simulink model "quadplane_control_conf"  (R2023a)
settings: Solver=FixedStepAuto  StartTime=0.0  StopTime=10.0  FixedStep=0.001  RelTol=1e-3
undefined symbols (not defined in the file or in its folder): Aircraft, DiscIntNeverNeededParam, framePeriod_s, frameRate_hz
libraries: simulink x14, fuzblock x1
(part 1 of 2)
settings Model: Creator=lagerprocessor  LastModifiedBy=abhandari1
settings DebuggingCC: ParameterPrecisionLossMsg=none

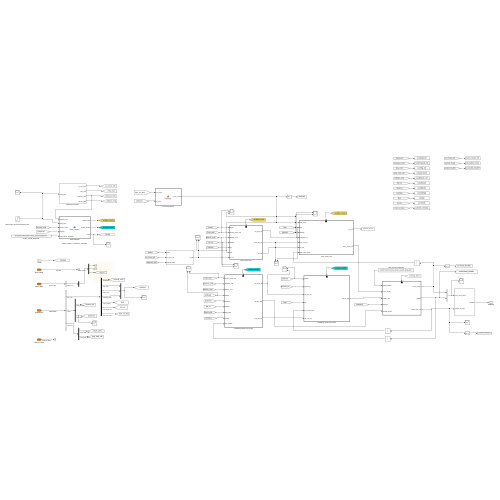
[thumbnail: Simulink's stored preview of the top-level diagram]
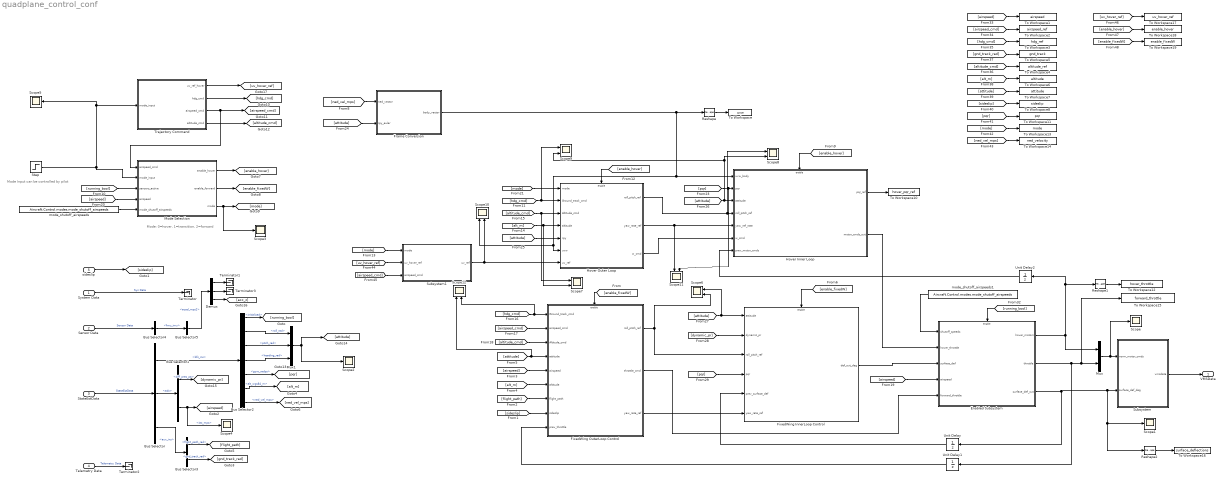
== system quadplane_control_conf ==
  note: Mode Input can be controlled by pilot
  note: Mode: 0=hover, 1=transition, 2=forward
  System Data : Inport  OutDataTypeStr=Bus: SysData  SampleTime=framePeriod_s  BusOutputAsStruct=on
  Sensor Data : Inport  Port=2  OutDataTypeStr=Bus: SensorData  SampleTime=framePeriod_s  BusOutputAsStruct=on
  StateEstData : Inport  Port=3  OutDataTypeStr=Bus: StateEstData  BusOutputAsStruct=on
  Telemetry Data : Inport  Port=4  OutDataTypeStr=Bus: TelemData  SampleTime=framePeriod_s  BusOutputAsStruct=on
  sideslip : Inport  Port=5  OutDataTypeStr=single
  Bus Selector : BusSelector  OutputSignals=bfs_ins,adc,aux_ins
  Bus Selector1 : BusSelector  OutputSignals=diff_pres_pa,ias_mps
  Bus Selector2 : BusSelector  OutputSignals=initialized,roll_rad,pitch_rad,heading_rad,gyro_radps,alt_wgs84_m,ned_vel_mps
  Bus Selector3 : BusSelector  OutputSignals=flight_path_rad,gnd_track_rad
  Bus Selector4 : BusSelector  OutputSignals=fmu_imu
  Bus Selector5 : BusSelector  OutputSignals=accel_mps2
  Demux : Demux  Outputs=3
  Enabled Subsystem : Subsystem  TreatAsAtomicUnit=on
  FixedWing InnerLoop Control : Subsystem  TreatAsAtomicUnit=on
  FixedWing OuterLoop Control : Subsystem  TreatAsAtomicUnit=on
  Frame Conversion : MATLAB Function  TreatAsAtomicUnit=on
  Hover Inner Loop : Subsystem  TreatAsAtomicUnit=on
  Hover Outer Loop : Subsystem  TreatAsAtomicUnit=on
  Mode Selection : MATLAB Function  TreatAsAtomicUnit=on
  Mux : Mux  Inputs=2
  Mux1 : Mux  Inputs=3
  Reshape : Reshape
  Reshape1 : Reshape
  Reshape2 : Reshape
  Scope{,1..5} (6 alike) : Scope
  Scope{6..12} (7 alike) : Scope  NumInputPorts=2
  Step : Step  Time=7  OutDataTypeStr=single  SampleTime=0
  Subsystem : Subsystem
  Subsystem1 : Subsystem
  Terminator{,1..3} (4 alike) : Terminator
  To Workspace : ToWorkspace  VariableName=uvw  SampleTime=-1
      settings: Save2DSignal=2-D array (concatenate along first dimension)
  To Workspace1 : ToWorkspace  VariableName=airspeed  SaveFormat=Timeseries  SampleTime=-1
  To Workspace10 : ToWorkspace  VariableName=hover_pqr_ref  SaveFormat=Timeseries  SampleTime=-1
  To Workspace11 : ToWorkspace  VariableName=pqr  SaveFormat=Timeseries  SampleTime=-1
  To Workspace12 : ToWorkspace  VariableName=hover_throttle  SampleTime=-1
      settings: Save2DSignal=2-D array (concatenate along first dimension)
  To Workspace13 : ToWorkspace  VariableName=mode  SaveFormat=Timeseries  SampleTime=-1
  To Workspace14 : ToWorkspace  VariableName=ned_velocity  SaveFormat=Timeseries  SampleTime=-1
  To Workspace15 : ToWorkspace  VariableName=forward_throttle  SaveFormat=Timeseries  SampleTime=-1
  To Workspace16 : ToWorkspace  VariableName=surface_deflections  SampleTime=-1
      settings: Save2DSignal=2-D array (concatenate along first dimension)
  To Workspace17 : ToWorkspace  VariableName=uv_hover_ref  SaveFormat=Timeseries  SampleTime=-1
  To Workspace18 : ToWorkspace  VariableName=enable_hover  SaveFormat=Timeseries  SampleTime=-1
  To Workspace19 : ToWorkspace  VariableName=enable_fixedW  SaveFormat=Timeseries  SampleTime=-1
  To Workspace2 : ToWorkspace  VariableName=airspeed_ref  SaveFormat=Timeseries  SampleTime=-1
  To Workspace3 : ToWorkspace  VariableName=hdg_ref  SaveFormat=Timeseries  SampleTime=-1
  To Workspace4 : ToWorkspace  VariableName=altitude_ref  SaveFormat=Timeseries  SampleTime=-1
  To Workspace5 : ToWorkspace  VariableName=gnd_track  SaveFormat=Timeseries  SampleTime=-1
  To Workspace6 : ToWorkspace  VariableName=altitude  SaveFormat=Timeseries  SampleTime=-1
  To Workspace7 : ToWorkspace  VariableName=attitude  SaveFormat=Timeseries  SampleTime=-1
  To Workspace8 : ToWorkspace  VariableName=sideslip  SaveFormat=Timeseries  SampleTime=-1
  Trajectory Command : Subsystem
  Unit Delay : UnitDelay  SampleTime=-1  HasFrameUpgradeWarning=on
  Unit Delay1 : UnitDelay  SampleTime=-1  HasFrameUpgradeWarning=on
  Unit Delay2 : UnitDelay  SampleTime=-1  HasFrameUpgradeWarning=on
  mode_shutoff_airspeeds : Constant  Value=Aircraft.Control.modes.mode_shutoff_airspeeds  OutDataTypeStr=single
  mode_shutoff_airspeeds1 : Constant  Value=Aircraft.Control.modes.mode_shutoff_airspeeds  OutDataTypeStr=single
  VMSData : Outport  OutDataTypeStr=Bus: VmsData
  wires:
  Telemetry Data/1 -> Terminator2/1  "Telemetry Data"
  StateEstData/1 -> Bus Selector/1  "StateEstData"
  Sensor Data/1 -> Bus Selector4/1  "Sensor Data"
  System Data/1 -> Terminator/1  "Sys Data"
  Subsystem/1(vmsdata) -> VMSData/1
  Bus Selector/2 -> Bus Selector1/1  "<adc>"
  Bus Selector/1 -> Bus Selector2/1  "<bfs_ins>"
  [enable_fixedW] -> FixedWing InnerLoop Control/Enable
  Bus Selector2/3 -> Mux1/2  "<pitch_rad>"
  Bus Selector2/4 -> Mux1/3  "<heading_rad>"
  Bus Selector/3 -> Bus Selector3/1  "<aux_ins>"
  Bus Selector4/1 -> Bus Selector5/1  "<fmu_imu>"
  Bus Selector5/1 -> Demux/1  "<accel_mps2>"
  Demux/1 -> Terminator1/1
  Demux/2 -> Terminator3/1
  sideslip/1 -> [sideslip]
  [sideslip] -> FixedWing OuterLoop Control/8(sideslip)
  Bus Selector2/1 -> [running_bool]  "<initialized>"
  Bus Selector2/2 -> Mux1/1  "<roll_rad>"
  [hdg_cmd] -> Scope12/2, FixedWing OuterLoop Control/1(Ground_track_cmd)
  Bus Selector3/2 -> [gnd_track_rad]  "<gnd_track_rad>"
  Bus Selector2/6 -> [alt_m]  "<alt_wgs84_m>"
  FixedWing OuterLoop Control/1(roll_pitch_ref) -> FixedWing InnerLoop Control/3(roll_pitch_ref), Scope6/2
  [airspeed_cmd] -> FixedWing OuterLoop Control/2(airspeed_cmd)
  [altitude_cmd] -> FixedWing OuterLoop Control/3(Altitude_cmd)
  [flight_path] -> FixedWing OuterLoop Control/7(flight_path)
  [airspeed] -> FixedWing OuterLoop Control/5(airspeed)
  [alt_m] -> FixedWing OuterLoop Control/6(altitude)
  [attitude] -> Scope12/1, FixedWing OuterLoop Control/4(attitude)
  [enable_fixedW] -> FixedWing OuterLoop Control/Enable
  Bus Selector2/7 -> [ned_vel_mps]  "<ned_vel_mps>"
  [ned_vel_mps] -> Frame Conversion/1(ned_vector)
  FixedWing OuterLoop Control/2(throttle_cmd) -> Enabled Subsystem/5(forward_throttle)
  FixedWing InnerLoop Control/1(def_out_deg) -> Enabled Subsystem/3(surface_def)
  [enable_hover] -> Hover Inner Loop/Enable
  Hover Inner Loop/2(motor_cmds_out) -> Enabled Subsystem/2(hover_throttle)
  Hover Outer Loop/1(roll_pitch_ref) -> Scope8/1, Hover Inner Loop/4(roll_pitch_ref)
  Hover Outer Loop/2(yaw_rate_ref) -> Hover Inner Loop/5(yaw_ref_rate), Scope11/1
  [enable_hover] -> Hover Outer Loop/Enable
  Hover Outer Loop/3(w_cmd) -> Hover Inner Loop/6(w_cmd)
  [hdg_cmd] -> Scope9/1, Hover Outer Loop/2(Ground_track_cmd)
  [altitude_cmd] -> Scope7/1, Hover Outer Loop/3(Altitude_cmd)
  [alt_m] -> Hover Outer Loop/4(altitude), Scope7/2
  Step/1 -> Mode Selection/2(mode_input), Scope5/1, Trajectory Command/1(mode_input)
  Mode Selection/1(enable_hover) -> [enable_hover]
  Mode Selection/2(enable_forward) -> [enable_fixedW]
  [running_bool] -> Mode Selection/3(sensors_active)
  Trajectory Command/2(hdg_cmd) -> [hdg_cmd]
  Trajectory Command/4(altitude_cmd) -> [altitude_cmd]
  Trajectory Command/3(airspeed_cmd) -> [airspeed_cmd], Mode Selection/1(airspeed_cmd)
  [airspeed] -> Enabled Subsystem/4(airspeed)
  Mux/1 -> Scope/1, Subsystem/1(norm_motor_cmds)
  Enabled Subsystem/2(throttle) -> Unit Delay1/1, To Workspace15/1, Mux/2
  Unit Delay/1 -> FixedWing InnerLoop Control/5(prev_surface_def)
  Unit Delay1/1 -> FixedWing OuterLoop Control/9(prev_throttle)
  Unit Delay2/1 -> Hover Inner Loop/7(prev_motor_cmds)
  [airspeed] -> Mode Selection/4(airspeed)
  mode_shutoff_airspeeds/1 -> Mode Selection/5(mode_shutoff_airspeeds)
  [mode] -> Hover Outer Loop/1(mode)
  Mode Selection/3(mode) -> Scope3/1, [mode]
  Bus Selector2/5 -> [pqr]  "<gyro_radps>"
  Mux1/1 -> Scope2/1, [attitude]
  Bus Selector1/1 -> [dynamic_pr]  "<diff_pres_pa>"
  Bus Selector3/1 -> [flight_path]  "<flight_path_rad>"
  Demux/3 -> [acc_z]
  [attitude] -> Frame Conversion/2(rpy_euler)
  [attitude] -> Hover Outer Loop/5(rpy)
  [pqr] -> Scope11/2, Hover Inner Loop/2(pqr)
  [attitude] -> Scope8/2, Scope9/2, Hover Inner Loop/3(attitude)
  [attitude] -> Scope6/1, FixedWing InnerLoop Control/1(attitude)
  [dynamic_pr] -> FixedWing InnerLoop Control/2(dynamic_pr)
  [pqr] -> FixedWing InnerLoop Control/4(pqr)
  mode_shutoff_airspeeds1/1 -> Enabled Subsystem/1(shutoff_speeds)
  Bus Selector1/2 -> Scope4/1, [airspeed]  "<ias_mps>"
  [running_bool] -> Enabled Subsystem/Enable
  Frame Conversion/1(body_vector) -> Reshape/1, Scope10/1, Hover Outer Loop/6(uvw), Hover Inner Loop/1(uvw_body)
  [airspeed] -> To Workspace1/1
  [airspeed_cmd] -> To Workspace2/1
  [hdg_cmd] -> To Workspace3/1
  [altitude_cmd] -> To Workspace4/1
  [gnd_track_rad] -> To Workspace5/1
  [alt_m] -> To Workspace6/1
  [attitude] -> To Workspace7/1
  [sideslip] -> To Workspace8/1
  Hover Inner Loop/1(pqr_ref) -> To Workspace10/1
  [pqr] -> To Workspace11/1
  [mode] -> To Workspace13/1
  [ned_vel_mps] -> To Workspace14/1
  Trajectory Command/1(uv_ref_hover) -> [uv_hover_ref]
  Reshape/1 -> To Workspace/1
  Enabled Subsystem/1(hover_motors) -> Mux/1, Reshape1/1, Unit Delay2/1
  Reshape1/1 -> To Workspace12/1
  Enabled Subsystem/3(surface_def_out) -> Scope1/1, Reshape2/1, Subsystem/2(surface_def_deg), Unit Delay/1
  Reshape2/1 -> To Workspace16/1
  Subsystem1/1(uv_ref) -> Scope10/2, Hover Outer Loop/7(uv_ref)
  [mode] -> Subsystem1/1(mode)
  [airspeed_cmd] -> Subsystem1/3(airspeed_cmd)
  [uv_hover_ref] -> Subsystem1/2(uv_hover_ref)
  [enable_hover] -> To Workspace18/1
  [enable_fixedW] -> To Workspace19/1
  [uv_hover_ref] -> To Workspace17/1
  FixedWing OuterLoop Control/3(yaw_rate_ref) -> FixedWing InnerLoop Control/6(yaw_rate_ref)

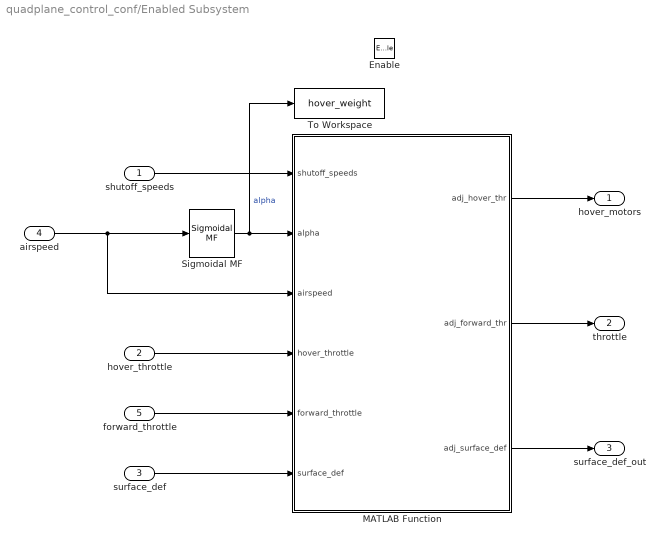
== system quadplane_control_conf/Enabled Subsystem ==
  shutoff_speeds : Inport
  hover_throttle : Inport  Port=2
  surface_def : Inport  Port=3
  airspeed : Inport  Port=4
  forward_throttle : Inport  Port=5
  Enable : EnablePort
  MATLAB Function : MATLAB Function  TreatAsAtomicUnit=on
  Sigmoidal MF : fuzblock/Membership  Functions/Sigmoidal MF  a=Aircraft.Control.modes.transition_sigmoidal_a  c=Aircraft.Control.modes.transition_sigmoidal_c
  To Workspace : ToWorkspace  VariableName=hover_weight  SaveFormat=Timeseries  SampleTime=-1
  hover_motors : Outport
  throttle : Outport  Port=2
  surface_def_out : Outport  Port=3
  wires:
  MATLAB Function/3(adj_surface_def) -> surface_def_out/1
  shutoff_speeds/1 -> MATLAB Function/1(shutoff_speeds)
  MATLAB Function/2(adj_forward_thr) -> throttle/1
  airspeed/1 -> MATLAB Function/3(airspeed), Sigmoidal MF/1
  forward_throttle/1 -> MATLAB Function/5(forward_throttle)
  surface_def/1 -> MATLAB Function/6(surface_def)
  Sigmoidal MF/1 -> To Workspace/1, MATLAB Function/2(alpha)  "alpha"
  MATLAB Function/1(adj_hover_thr) -> hover_motors/1
  hover_throttle/1 -> MATLAB Function/4(hover_throttle)

== system quadplane_control_conf/FixedWing InnerLoop Control ==
  attitude : Inport
  dynamic_pr : Inport  Port=2
  roll_pitch_ref : Inport  Port=3
  pqr : Inport  Port=4
  prev_surface_def : Inport  Port=5
  yaw_rate_ref : Inport  Port=6
  Enable : EnablePort
  INDI Based Angular Rate Controller : Subsystem
  NDI based Attitude Controller : Subsystem
  def_out_deg : Outport
  wires:
  dynamic_pr/1 -> INDI Based Angular Rate Controller/1(dynamic_pr)
  pqr/1 -> INDI Based Angular Rate Controller/3(pqr)
  attitude/1 -> NDI based Attitude Controller/1(attitude)
  NDI based Attitude Controller/1(pqr_ref) -> INDI Based Angular Rate Controller/2(pqr_ref)
  roll_pitch_ref/1 -> NDI based Attitude Controller/2(roll_pitch_ref)
  prev_surface_def/1 -> INDI Based Angular Rate Controller/4(prev_surface_def)
  INDI Based Angular Rate Controller/1(def_out_deg) -> def_out_deg/1
  yaw_rate_ref/1 -> NDI based Attitude Controller/3(yaw_rate_ref)

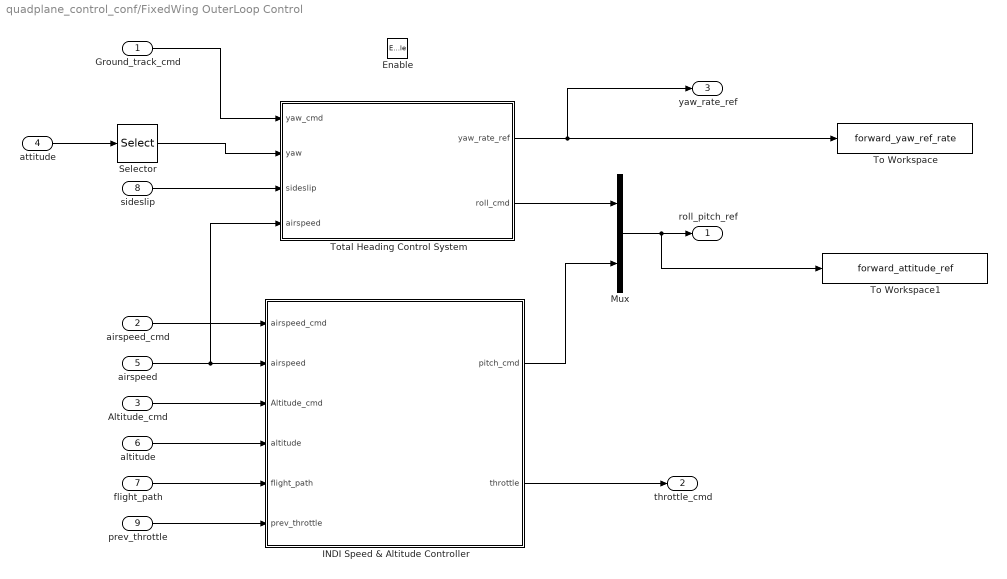
== system quadplane_control_conf/FixedWing OuterLoop Control ==
  Ground_track_cmd : Inport
  airspeed_cmd : Inport  Port=2
  Altitude_cmd : Inport  Port=3
  attitude : Inport  Port=4
  airspeed : Inport  Port=5
  altitude : Inport  Port=6
  flight_path : Inport  Port=7
  sideslip : Inport  Port=8
  prev_throttle : Inport  Port=9
  Enable : EnablePort
  INDI Speed & Altitude Controller : Subsystem
  Mux : Mux  Inputs=2
  Selector : Selector  InputPortWidth=3  IndexOptions=Index vector (dialog)  Indices=3  OutputSizes=1
  To Workspace : ToWorkspace  VariableName=forward_yaw_ref_rate  SaveFormat=Timeseries  SampleTime=-1
  To Workspace1 : ToWorkspace  VariableName=forward_attitude_ref  SaveFormat=Timeseries  SampleTime=-1
  Total Heading Control System : Subsystem
  roll_pitch_ref : Outport
  throttle_cmd : Outport  Port=2
  yaw_rate_ref : Outport  Port=3
  wires:
  Ground_track_cmd/1 -> Total Heading Control System/1(yaw_cmd)
  Altitude_cmd/1 -> INDI Speed & Altitude Controller/3(Altitude_cmd)
  INDI Speed & Altitude Controller/2(throttle) -> throttle_cmd/1
  altitude/1 -> INDI Speed & Altitude Controller/4(altitude)
  flight_path/1 -> INDI Speed & Altitude Controller/5(flight_path)
  INDI Speed & Altitude Controller/1(pitch_cmd) -> Mux/2
  airspeed_cmd/1 -> INDI Speed & Altitude Controller/1(airspeed_cmd)
  Total Heading Control System/2(roll_cmd) -> Mux/1
  airspeed/1 -> Total Heading Control System/4(airspeed), INDI Speed & Altitude Controller/2(airspeed)
  Selector/1 -> Total Heading Control System/2(yaw)
  prev_throttle/1 -> INDI Speed & Altitude Controller/6(prev_throttle)
  Mux/1 -> To Workspace1/1, roll_pitch_ref/1
  attitude/1 -> Selector/1
  sideslip/1 -> Total Heading Control System/3(sideslip)
  Total Heading Control System/1(yaw_rate_ref) -> yaw_rate_ref/1, To Workspace/1

== system quadplane_control_conf/Hover Inner Loop ==
  uvw_body : Inport
  pqr : Inport  Port=2
  attitude : Inport  Port=3
  roll_pitch_ref : Inport  Port=4
  yaw_ref_rate : Inport  Port=5
  w_cmd : Inport  Port=6
  prev_motor_cmds : Inport  Port=7
  Enable : EnablePort
  Attitude Control : Subsystem
  INDI inner loop : Subsystem
  pqr_ref : Outport
  motor_cmds_out : Outport  Port=2
  wires:
  Attitude Control/1(pqr_ref1) -> pqr_ref/1, INDI inner loop/1(pqr_ref)
  uvw_body/1 -> INDI inner loop/2(uvw_body)
  pqr/1 -> INDI inner loop/4(pqr)
  INDI inner loop/1(motor_cmds_out) -> motor_cmds_out/1
  attitude/1 -> Attitude Control/3(roll_pitch_yaw)
  yaw_ref_rate/1 -> Attitude Control/1(yaw_rate_ref)
  roll_pitch_ref/1 -> Attitude Control/2(roll_pitch_ref)
  w_cmd/1 -> INDI inner loop/3(w_ref)
  prev_motor_cmds/1 -> INDI inner loop/5(prev_motor_cmds)

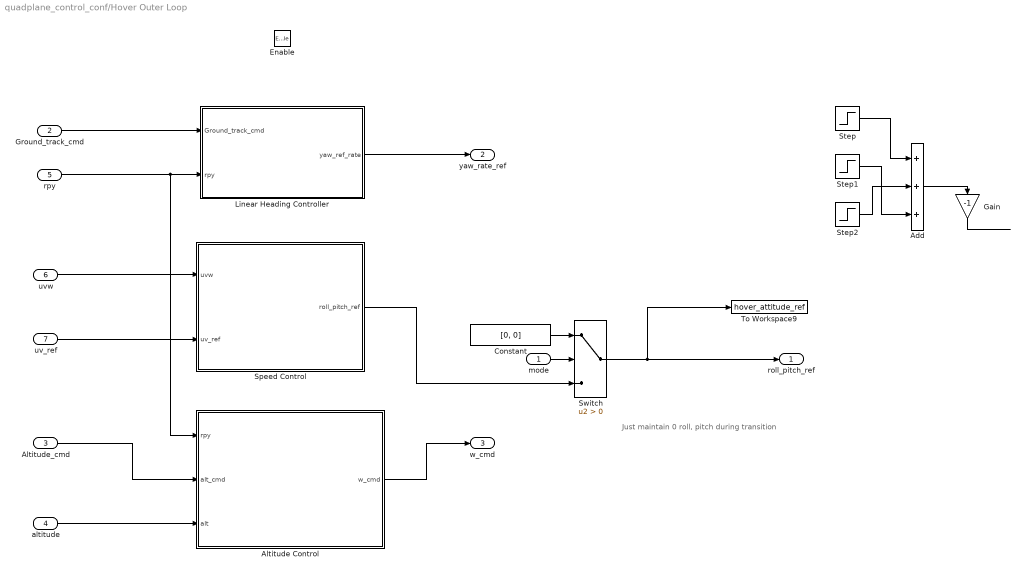
== system quadplane_control_conf/Hover Outer Loop ==
  note: Just maintain 0 roll, pitch during transition
  mode : Inport
  Ground_track_cmd : Inport  Port=2
  Altitude_cmd : Inport  Port=3
  altitude : Inport  Port=4
  rpy : Inport  Port=5
  uvw : Inport  Port=6
  uv_ref : Inport  Port=7
  Enable : EnablePort
  Add : Sum  Inputs=+++
  Altitude Control : Subsystem
  Constant : Constant  Value=[0, 0]  OutDataTypeStr=single
  Gain : Gain  Gain=-1
  Linear Heading Controller : Subsystem
  Speed Control : Subsystem
  Step : Step  Time=2  After=0.5  OutDataTypeStr=single  SampleTime=0
  Step1 : Step  Time=4  Before=0.5  After=-0.5  OutDataTypeStr=single  SampleTime=0
  Step2 : Step  Time=7  Before=-0.5  After=0  OutDataTypeStr=single  SampleTime=0
  Switch : Switch  Criteria=u2 > Threshold  SaturateOnIntegerOverflow=off  InputSameDT=off
  To Workspace9 : ToWorkspace  VariableName=hover_attitude_ref  SaveFormat=Timeseries  SampleTime=-1
  roll_pitch_ref : Outport
  yaw_rate_ref : Outport  Port=2
  w_cmd : Outport  Port=3
  wires:
  Ground_track_cmd/1 -> Linear Heading Controller/1(Ground_track_cmd)
  Altitude_cmd/1 -> Altitude Control/2(alt_cmd)
  altitude/1 -> Altitude Control/3(alt)
  rpy/1 -> Altitude Control/1(rpy), Linear Heading Controller/2(rpy)
  uvw/1 -> Speed Control/1(uvw)
  Speed Control/1(roll_pitch_ref) -> Switch/3
  Altitude Control/1(w_cmd) -> w_cmd/1
  Switch/1 -> To Workspace9/1, roll_pitch_ref/1
  mode/1 -> Switch/2
  Constant/1 -> Switch/1
  uv_ref/1 -> Speed Control/2(uv_ref)
  Step/1 -> Add/1
  Step1/1 -> Add/3
  Step2/1 -> Add/2
  Add/1 -> Gain/1
  Gain/1 -> ?
  Linear Heading Controller/1(yaw_ref_rate) -> yaw_rate_ref/1

== system quadplane_control_conf/Subsystem ==
  note: norm_motor_cmds = [0,1]
  note: surface_def = [-30, 30]
  norm_motor_cmds : Inport
  surface_def_deg : Inport  Port=2
  Subsystem1 : Subsystem
  deflections_PWM_denormalize : Subsystem
  motor_PWM_denormalize : Subsystem
  vmsdata : Outport
  wires:
  motor_PWM_denormalize/1(raw_output) -> Subsystem1/1(Motor_Cmds)
  deflections_PWM_denormalize/1(raw_output) -> Subsystem1/2(Surface_def)
  Subsystem1/1(vmsdata) -> vmsdata/1
  norm_motor_cmds/1 -> motor_PWM_denormalize/1(normalized_input)
  surface_def_deg/1 -> deflections_PWM_denormalize/1(normalized_input)

== system quadplane_control_conf/Subsystem1 ==
  mode : Inport
  uv_hover_ref : Inport  Port=2
  airspeed_cmd : Inport  Port=3
  Constant : Constant  Value=0  OutDataTypeStr=single
  Mux : Mux  Inputs=2
  Switch : Switch  Criteria=u2 > Threshold  SaturateOnIntegerOverflow=off  InputSameDT=off
  uv_ref : Outport
  wires:
  Switch/1 -> uv_ref/1
  mode/1 -> Switch/2
  airspeed_cmd/1 -> Mux/1
  Constant/1 -> Mux/2
  Mux/1 -> Switch/1
  uv_hover_ref/1 -> Switch/3

== system quadplane_control_conf/Trajectory Command ==
  mode_input : Inport
  Subsystem : Subsystem
  Subsystem1 : Subsystem
  Subsystem2 : Subsystem
  Subsystem3 : Subsystem
  uv_ref_hover : Outport
  hdg_cmd : Outport  Port=2
  airspeed_cmd : Outport  Port=3
  altitude_cmd : Outport  Port=4
  wires:
  Subsystem/1(uv_ref_hover) -> uv_ref_hover/1
  Subsystem1/1(hdg_cmd) -> hdg_cmd/1
  Subsystem2/1(airspeed_cmd) -> airspeed_cmd/1
  Subsystem3/1(altitude_cmd) -> altitude_cmd/1
  mode_input/1 -> Subsystem2/1(mode_input)

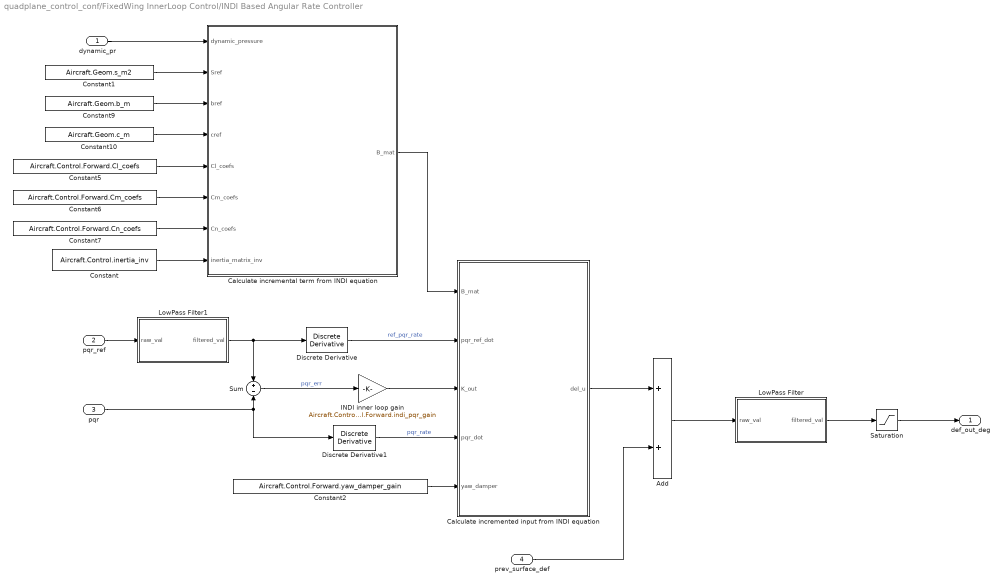
== system quadplane_control_conf/FixedWing InnerLoop Control/INDI Based Angular Rate Controller ==
  dynamic_pr : Inport
  pqr_ref : Inport  Port=2
  pqr : Inport  Port=3
  prev_surface_def : Inport  Port=4
  Add : Sum  OutDataTypeStr=single
  Calculate incremental term from INDI equation : MATLAB Function  TreatAsAtomicUnit=on
  Calculate incremented input from INDI equation : MATLAB Function  TreatAsAtomicUnit=on
  Constant : Constant  Value=Aircraft.Control.inertia_inv  OutDataTypeStr=single
  Constant1 : Constant  Value=Aircraft.Geom.s_m2  OutDataTypeStr=single
  Constant10 : Constant  Value=Aircraft.Geom.c_m  OutDataTypeStr=single
  Constant2 : Constant  Value=Aircraft.Control.Forward.yaw_damper_gain  OutDataTypeStr=single
  Constant5 : Constant  Value=Aircraft.Control.Forward.Cl_coefs  OutDataTypeStr=single
  Constant6 : Constant  Value=Aircraft.Control.Forward.Cm_coefs  OutDataTypeStr=single
  Constant7 : Constant  Value=Aircraft.Control.Forward.Cn_coefs  OutDataTypeStr=single
  Constant9 : Constant  Value=Aircraft.Geom.b_m  OutDataTypeStr=single
  Discrete Derivative : simulink/Discrete/Discrete Derivative  gainval=1.0  ICPrevScaledInput=0.0  OutMin=[]  OutMax=[]  OutDataTypeStr=single  OutputDataTypeScalingMode=single  OutDataType=fixdt(1, 16)  OutScaling=2^-10  DoSatur=off
  Discrete Derivative1 : simulink/Discrete/Discrete Derivative  gainval=1.0  ICPrevScaledInput=0.0  OutMin=[]  OutMax=[]  OutDataType=fixdt(1, 16)  OutScaling=2^-10  DoSatur=off
  INDI inner loop gain : Gain  Gain=Aircraft.Control.Forward.indi_pqr_gain  OutDataTypeStr=single
  LowPass Filter : Subsystem
      settings: PortSchema="{\"entries\":[{\"content\":{\"sides\":[{\"content\":{\"connectorIds\":[\"Out1\"]},\"type\":\"ConnectorPlacement.EquallySpacedRectSide\",\"uuid\":\"91cc3e13-2b14-472d-8884-d1975898cd34\"},{\"content\":{\"connectorIds\":[\"In1\"],\"side\":\"RIGHT\"},\"type\":\"ConnectorPlacement.EquallySpacedRectSide\",\"uuid\":\"ce6b3021-6e32-4737-8c8e-25014706d3dd\"},{\"content\":{\"side\":\"TOP\"},\"type\":\"ConnectorPlacement.EquallySpacedRectSide\",\"uuid\":\"ad734f0b-b067-43e6-a641-0e0955250a7f\"},{\"content\":{\"side\":\"BOTTOM\"},\"type\":\"ConnectorPlacement.EquallySpacedRectSide\",\"uuid\":\"618c62c8-d4e2-4678-9fe1-905e2f147d5d\"}]},\"type\":\"ConnectorPlacement.EquallySpacedConnector\",\"uuid\":\"c0097053-d36a-473a-84fb-0616f69f4bc5\"}],\"packageUris\":[\"http://schema.mathworks.com/mf0/Connector/R2020b\"],\"version\":\"1.0\"}"
  LowPass Filter1 : Subsystem
      settings: PortSchema="{\"entries\":[{\"content\":{\"sides\":[{\"content\":{\"connectorIds\":[\"Out1\"]},\"type\":\"ConnectorPlacement.EquallySpacedRectSide\",\"uuid\":\"91cc3e13-2b14-472d-8884-d1975898cd34\"},{\"content\":{\"connectorIds\":[\"In1\"],\"side\":\"RIGHT\"},\"type\":\"ConnectorPlacement.EquallySpacedRectSide\",\"uuid\":\"ce6b3021-6e32-4737-8c8e-25014706d3dd\"},{\"content\":{\"side\":\"TOP\"},\"type\":\"ConnectorPlacement.EquallySpacedRectSide\",\"uuid\":\"ad734f0b-b067-43e6-a641-0e0955250a7f\"},{\"content\":{\"side\":\"BOTTOM\"},\"type\":\"ConnectorPlacement.EquallySpacedRectSide\",\"uuid\":\"618c62c8-d4e2-4678-9fe1-905e2f147d5d\"}]},\"type\":\"ConnectorPlacement.EquallySpacedConnector\",\"uuid\":\"c0097053-d36a-473a-84fb-0616f69f4bc5\"}],\"packageUris\":[\"http://schema.mathworks.com/mf0/Connector/R2020b\"],\"version\":\"1.0\"}"
  Saturation : Saturate  UpperLimit=Aircraft.Surf.Limit.pos_deg  LowerLimit=Aircraft.Surf.Limit.neg_deg  OutDataTypeStr=single
  Sum : Sum  Inputs=+-
  def_out_deg : Outport
  wires:
  Discrete Derivative1/1 -> Calculate incremented input from INDI equation/4(pqr_dot)  "pqr_rate"
  Constant2/1 -> Calculate incremented input from INDI equation/5(yaw_damper)
  Constant7/1 -> Calculate incremental term from INDI equation/7(Cn_coefs)
  Discrete Derivative/1 -> Calculate incremented input from INDI equation/2(pqr_ref_dot)  "ref_pqr_rate"
  Saturation/1 -> def_out_deg/1
  dynamic_pr/1 -> Calculate incremental term from INDI equation/1(dynamic_pressure)
  Constant1/1 -> Calculate incremental term from INDI equation/2(Sref)
  Constant10/1 -> Calculate incremental term from INDI equation/4(cref)
  Calculate incremented input from INDI equation/1(del_u) -> Add/1
  Constant6/1 -> Calculate incremental term from INDI equation/6(Cm_coefs)
  Sum/1 -> INDI inner loop gain/1  "pqr_err"
  INDI inner loop gain/1 -> Calculate incremented input from INDI equation/3(K_out)
  pqr/1 -> Discrete Derivative1/1, Sum/2
  Constant5/1 -> Calculate incremental term from INDI equation/5(Cl_coefs)
  Constant/1 -> Calculate incremental term from INDI equation/8(inertia_matrix_inv)
  Constant9/1 -> Calculate incremental term from INDI equation/3(bref)
  Calculate incremental term from INDI equation/1(B_mat) -> Calculate incremented input from INDI equation/1(B_mat)
  Add/1 -> LowPass Filter/1(raw_val)
  LowPass Filter/1(filtered_val) -> Saturation/1
  LowPass Filter1/1(filtered_val) -> Sum/1, Discrete Derivative/1
  prev_surface_def/1 -> Add/2
  pqr_ref/1 -> LowPass Filter1/1(raw_val)

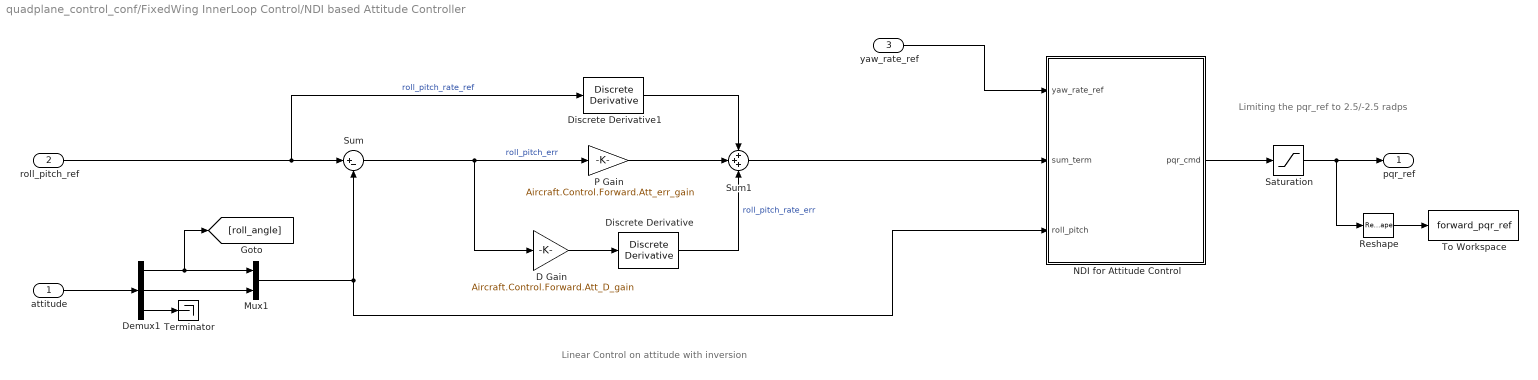
== system quadplane_control_conf/FixedWing InnerLoop Control/NDI based Attitude Controller ==
  note: Linear Control on attitude with inversion
  note: Limiting the pqr_ref to 2.5/-2.5 radps
  attitude : Inport
  roll_pitch_ref : Inport  Port=2
  yaw_rate_ref : Inport  Port=3
  D Gain : Gain  Gain=Aircraft.Control.Forward.Att_D_gain
  Demux1 : Demux  Outputs=3
  Discrete Derivative : simulink/Discrete/Discrete Derivative  gainval=1.0  ICPrevScaledInput=0.0  OutMin=[]  OutMax=[]  OutDataTypeStr=single  OutputDataTypeScalingMode=single  OutDataType=fixdt(1, 16)  OutScaling=2^-10  DoSatur=off
  Discrete Derivative1 : simulink/Discrete/Discrete Derivative  gainval=1.0  ICPrevScaledInput=0.0  OutMin=[]  OutMax=[]  OutDataTypeStr=single  OutputDataTypeScalingMode=single  OutDataType=fixdt(1, 16)  OutScaling=2^-10  DoSatur=off
  Mux1 : Mux  Inputs=2
  NDI for Attitude Control : MATLAB Function  TreatAsAtomicUnit=on
  P Gain : Gain  Gain=Aircraft.Control.Forward.Att_err_gain  OutDataTypeStr=single
  Reshape : Reshape
  Saturation : Saturate  UpperLimit=Aircraft.Control.Forward.max_pqr_ref  LowerLimit=-Aircraft.Control.Forward.max_pqr_ref
  Sum : Sum  Inputs=|+-  AccumDataTypeStr=single
  Sum1 : Sum  Inputs=+++  OutDataTypeStr=single
  Terminator : Terminator
  To Workspace : ToWorkspace  VariableName=forward_pqr_ref  SaveFormat=Timeseries  SampleTime=-1
  pqr_ref : Outport
  wires:
  Sum/1 -> D Gain/1, P Gain/1  "roll_pitch_err"
  Discrete Derivative1/1 -> Sum1/1
  P Gain/1 -> Sum1/2
  Discrete Derivative/1 -> Sum1/3  "roll_pitch_rate_err"
  Demux1/1 -> [roll_angle], Mux1/1
  attitude/1 -> Demux1/1
  Demux1/3 -> Terminator/1
  Demux1/2 -> Mux1/2
  Mux1/1 -> Sum/2, NDI for Attitude Control/3(roll_pitch)
  D Gain/1 -> Discrete Derivative/1
  NDI for Attitude Control/1(pqr_cmd) -> Saturation/1
  Sum1/1 -> NDI for Attitude Control/2(sum_term)
  Saturation/1 -> Reshape/1, pqr_ref/1
  roll_pitch_ref/1 -> Discrete Derivative1/1, Sum/1  "roll_pitch_rate_ref"
  yaw_rate_ref/1 -> NDI for Attitude Control/1(yaw_rate_ref)
  Reshape/1 -> To Workspace/1

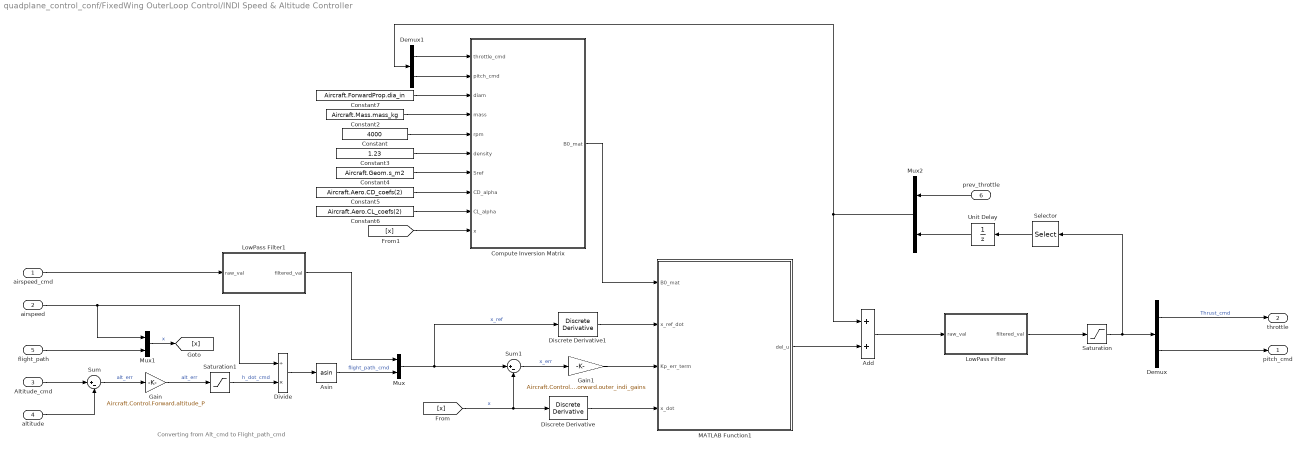
== system quadplane_control_conf/FixedWing OuterLoop Control/INDI Speed & Altitude Controller ==
  note: Converting from Alt_cmd to Flight_path_cmd
  airspeed_cmd : Inport
  airspeed : Inport  Port=2
  Altitude_cmd : Inport  Port=3
  altitude : Inport  Port=4
  flight_path : Inport  Port=5
  prev_throttle : Inport  Port=6
  Add : Sum  OutDataTypeStr=single
  Asin : Trigonometry  Operator=asin
  Compute Inversion Matrix : MATLAB Function  TreatAsAtomicUnit=on
  Constant : Constant  Value=4000  OutDataTypeStr=single
  Constant2 : Constant  Value=Aircraft.Mass.mass_kg  OutDataTypeStr=single
  Constant3 : Constant  Value=1.23  OutDataTypeStr=single
  Constant4 : Constant  Value=Aircraft.Geom.s_m2  OutDataTypeStr=single
  Constant5 : Constant  Value=Aircraft.Aero.CD_coefs(2)  OutDataTypeStr=single
  Constant6 : Constant  Value=Aircraft.Aero.CL_coefs(2)  OutDataTypeStr=single
  Constant7 : Constant  Value=Aircraft.ForwardProp.dia_in  OutDataTypeStr=single
  Demux : Demux  Outputs=2
  Demux1 : Demux  Outputs=2
  Discrete Derivative : simulink/Discrete/Discrete Derivative  gainval=1.0  ICPrevScaledInput=0.0  OutMin=[]  OutMax=[]  OutDataType=fixdt(1, 16)  OutScaling=2^-10  DoSatur=off
  Discrete Derivative1 : simulink/Discrete/Discrete Derivative  gainval=1.0  ICPrevScaledInput=0.0  OutMin=[]  OutMax=[]  OutDataType=fixdt(1, 16)  OutScaling=2^-10  DoSatur=off
  Divide : Product  Inputs=/*
  Gain : Gain  Gain=Aircraft.Control.Forward.altitude_P
  Gain1 : Gain  Gain=Aircraft.Control.Forward.outer_indi_gains
  LowPass Filter : Subsystem
  LowPass Filter1 : Subsystem
      settings: PortSchema="{\"entries\":[{\"content\":{\"sides\":[{\"content\":{\"connectorIds\":[\"Out1\"]},\"type\":\"ConnectorPlacement.EquallySpacedRectSide\",\"uuid\":\"91cc3e13-2b14-472d-8884-d1975898cd34\"},{\"content\":{\"connectorIds\":[\"In1\"],\"side\":\"RIGHT\"},\"type\":\"ConnectorPlacement.EquallySpacedRectSide\",\"uuid\":\"ce6b3021-6e32-4737-8c8e-25014706d3dd\"},{\"content\":{\"side\":\"TOP\"},\"type\":\"ConnectorPlacement.EquallySpacedRectSide\",\"uuid\":\"ad734f0b-b067-43e6-a641-0e0955250a7f\"},{\"content\":{\"side\":\"BOTTOM\"},\"type\":\"ConnectorPlacement.EquallySpacedRectSide\",\"uuid\":\"618c62c8-d4e2-4678-9fe1-905e2f147d5d\"}]},\"type\":\"ConnectorPlacement.EquallySpacedConnector\",\"uuid\":\"c0097053-d36a-473a-84fb-0616f69f4bc5\"}],\"packageUris\":[\"http://schema.mathworks.com/mf0/Connector/R2020b\"],\"version\":\"1.0\"}"
  MATLAB Function1 : MATLAB Function  TreatAsAtomicUnit=on
  Mux : Mux  Inputs=2
  Mux1 : Mux  Inputs=2
  Mux2 : Mux  Inputs=2
  Saturation : Saturate  UpperLimit=[1, Aircraft.Control.Forward.max_pitch_rad]'  LowerLimit=[0, -Aircraft.Control.Forward.max_pitch_rad]'
  Saturation1 : Saturate  UpperLimit=3  LowerLimit=-3
  Selector : Selector  InputPortWidth=2  IndexOptions=Index vector (dialog)  Indices=2  OutputSizes=1
  Sum : Sum  Inputs=|+-
  Sum1 : Sum  Inputs=|+-
  Unit Delay : UnitDelay  SampleTime=-1  HasFrameUpgradeWarning=on
  pitch_cmd : Outport
  throttle : Outport  Port=2
  wires:
  Altitude_cmd/1 -> Sum/1
  altitude/1 -> Sum/2
  Gain/1 -> Saturation1/1  "alt_err"
  airspeed_cmd/1 -> LowPass Filter1/1(raw_val)
  airspeed/1 -> Mux1/1, Divide/1
  Mux/1 -> Sum1/1, Discrete Derivative1/1  "x_ref"
  Mux1/1 -> [x]  "x"
  [x] -> Sum1/2, Discrete Derivative/1  "x"
  Sum1/1 -> Gain1/1  "x_err"
  Gain1/1 -> MATLAB Function1/3(Kp_err_term)
  Constant2/1 -> Compute Inversion Matrix/4(mass)
  Constant3/1 -> Compute Inversion Matrix/6(density)
  Constant4/1 -> Compute Inversion Matrix/7(Sref)
  Constant6/1 -> Compute Inversion Matrix/9(CL_alpha)
  Constant5/1 -> Compute Inversion Matrix/8(CD_alpha)
  [x] -> Compute Inversion Matrix/10(x)
  flight_path/1 -> Mux1/2
  Divide/1 -> Asin/1
  Asin/1 -> Mux/2  "flight_path_cmd"
  MATLAB Function1/1(del_u) -> Add/2
  Discrete Derivative/1 -> MATLAB Function1/4(x_dot)
  Demux/2 -> pitch_cmd/1
  Constant7/1 -> Compute Inversion Matrix/3(diam)
  Demux1/1 -> Compute Inversion Matrix/1(throttle_cmd)
  Demux1/2 -> Compute Inversion Matrix/2(pitch_cmd)
  Demux/1 -> throttle/1  "Thrust_cmd"
  Compute Inversion Matrix/1(B0_mat) -> MATLAB Function1/1(B0_mat)
  Saturation/1 -> Selector/1, Demux/1
  Discrete Derivative1/1 -> MATLAB Function1/2(x_ref_dot)
  Saturation1/1 -> Divide/2  "h_dot_cmd"
  Sum/1 -> Gain/1  "alt_err"
  Add/1 -> LowPass Filter/1(raw_val)
  LowPass Filter/1(filtered_val) -> Saturation/1
  LowPass Filter1/1(filtered_val) -> Mux/1
  Unit Delay/1 -> Mux2/2
  prev_throttle/1 -> Mux2/1
  Mux2/1 -> Demux1/1, Add/1
  Selector/1 -> Unit Delay/1
  Constant/1 -> Compute Inversion Matrix/5(rpm)

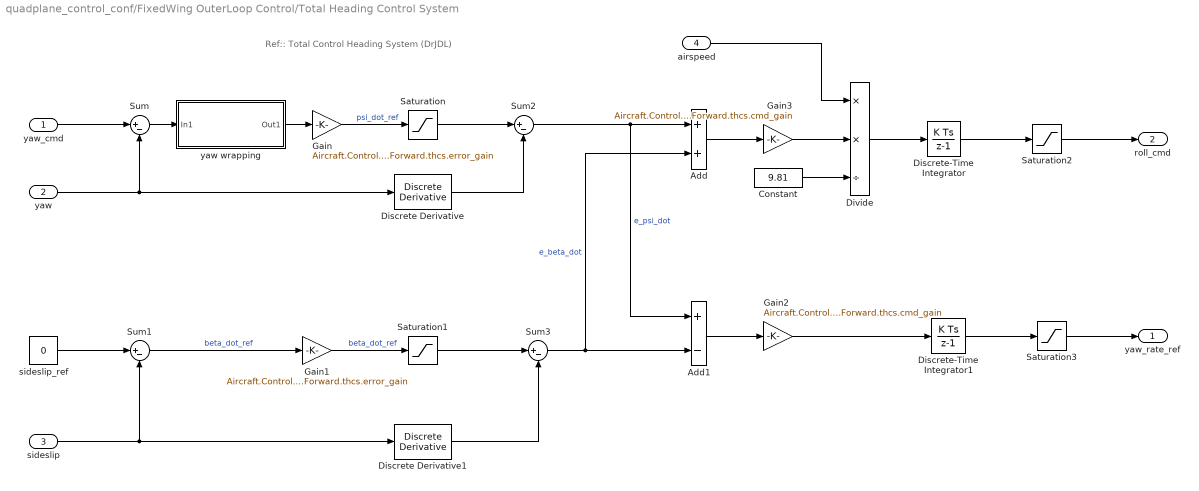
== system quadplane_control_conf/FixedWing OuterLoop Control/Total Heading Control System ==
  note: Ref:: Total Control Heading System (DrJDL)
  yaw_cmd : Inport
  yaw : Inport  Port=2
  sideslip : Inport  Port=3
  airspeed : Inport  Port=4
  " yaw wrapping" : Subsystem
  Add : Sum
  Add1 : Sum  Inputs=+-
  Constant : Constant  Value=9.81  OutDataTypeStr=single
  Discrete Derivative : simulink/Discrete/Discrete Derivative  gainval=1.0  ICPrevScaledInput=0.0  OutMin=[]  OutMax=[]  OutDataType=fixdt(1, 16)  OutScaling=2^-10  DoSatur=off
  Discrete Derivative1 : simulink/Discrete/Discrete Derivative  gainval=1.0  ICPrevScaledInput=0.0  OutMin=[]  OutMax=[]  OutDataType=fixdt(1, 16)  OutScaling=2^-10  DoSatur=off
  Discrete-Time Integrator : DiscreteIntegrator  SampleTime=-1  ICPrevOutput=DiscIntNeverNeededParam  ICPrevScaledInput=DiscIntNeverNeededParam
  Discrete-Time Integrator1 : DiscreteIntegrator  SampleTime=-1  ICPrevOutput=DiscIntNeverNeededParam  ICPrevScaledInput=DiscIntNeverNeededParam
  Divide : Product  Inputs=**/
  Gain : Gain  Gain=Aircraft.Control.Forward.thcs.error_gain
  Gain1 : Gain  Gain=Aircraft.Control.Forward.thcs.error_gain
  Gain2 : Gain  Gain=Aircraft.Control.Forward.thcs.cmd_gain
  Gain3 : Gain  Gain=Aircraft.Control.Forward.thcs.cmd_gain
  Saturation : Saturate  UpperLimit=Aircraft.Control.Forward.thcs.psi_dot_ref  LowerLimit=-Aircraft.Control.Forward.thcs.psi_dot_ref  OutDataTypeStr=single
  Saturation1 : Saturate  UpperLimit=Aircraft.Control.Forward.thcs.beta_dot_ref_limit  LowerLimit=-Aircraft.Control.Forward.thcs.beta_dot_ref_limit  OutDataTypeStr=single
  Saturation2 : Saturate  UpperLimit=Aircraft.Control.Forward.max_roll_rad  LowerLimit=-Aircraft.Control.Forward.max_roll_rad  OutDataTypeStr=single
  Saturation3 : Saturate  UpperLimit=Aircraft.Control.Forward.max_yaw_rate  LowerLimit=-Aircraft.Control.Forward.max_yaw_rate  OutDataTypeStr=single
  Sum{,1..3} (4 alike) : Sum  Inputs=|+-
  sideslip_ref : Constant  Value=0  OutDataTypeStr=single
  yaw_rate_ref : Outport
  roll_cmd : Outport  Port=2
  wires:
  yaw_cmd/1 -> Sum/1
  yaw/1 -> Sum/2, Discrete Derivative/1
  Sum/1 -> " yaw wrapping"/1(In1)
  sideslip_ref/1 -> Sum1/1
  sideslip/1 -> Sum1/2, Discrete Derivative1/1
  Gain/1 -> Saturation/1  "psi_dot_ref"
  Gain1/1 -> Saturation1/1  "beta_dot_ref"
  Saturation/1 -> Sum2/1
  Discrete Derivative/1 -> Sum2/2
  Sum2/1 -> Add1/1, Add/1  "e_psi_dot"
  Saturation1/1 -> Sum3/1
  Discrete Derivative1/1 -> Sum3/2
  Sum3/1 -> Add/2, Add1/2  "e_beta_dot"
  Add1/1 -> Gain2/1
  Gain2/1 -> Discrete-Time Integrator1/1
  Discrete-Time Integrator1/1 -> Saturation3/1
  Add/1 -> Gain3/1
  Gain3/1 -> Divide/2
  Constant/1 -> Divide/3
  Divide/1 -> Discrete-Time Integrator/1
  airspeed/1 -> Divide/1
  Discrete-Time Integrator/1 -> Saturation2/1
  " yaw wrapping"/1(Out1) -> Gain/1
  Saturation2/1 -> roll_cmd/1
  Saturation3/1 -> yaw_rate_ref/1
  Sum1/1 -> Gain1/1  "beta_dot_ref"

== system quadplane_control_conf/Hover Inner Loop/Attitude Control ==
  note: Limiting the pqr_ref to 2/-2 radps
  yaw_rate_ref : Inport
  roll_pitch_ref : Inport  Port=2
  roll_pitch_yaw : Inport  Port=3
  Gain : Gain  Gain=Aircraft.Control.Hover.att_gain
  Mux : Mux  Inputs=2
  Saturation : Saturate  UpperLimit=Aircraft.Control.Hover.pqr_limit  LowerLimit=-Aircraft.Control.Hover.pqr_limit
  Selector : Selector  InputPortWidth=3  IndexOptions=Index vector (dialog)  Indices=[1 2]  OutputSizes=1
  Sum : Sum  Inputs=|+-  AccumDataTypeStr=single
  pqr_ref1 : Outport
  wires:
  roll_pitch_ref/1 -> Sum/1
  Sum/1 -> Gain/1  "roll_pitch_err"
  Mux/1 -> Saturation/1
  Saturation/1 -> pqr_ref1/1
  yaw_rate_ref/1 -> Mux/2
  Selector/1 -> Sum/2
  roll_pitch_yaw/1 -> Selector/1
  Gain/1 -> Mux/1

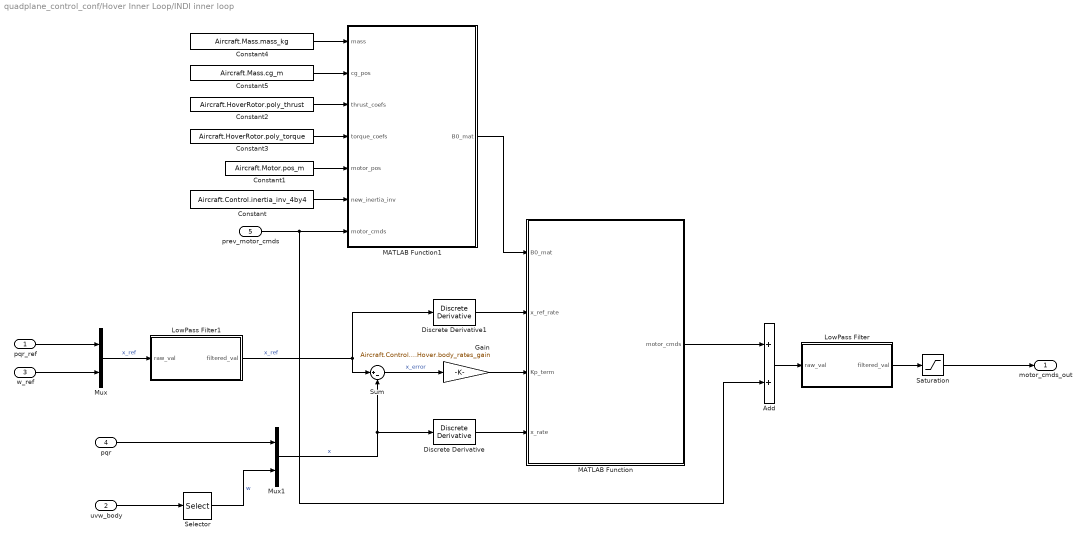
== system quadplane_control_conf/Hover Inner Loop/INDI inner loop ==
  pqr_ref : Inport
  uvw_body : Inport  Port=2
  w_ref : Inport  Port=3
  pqr : Inport  Port=4
  prev_motor_cmds : Inport  Port=5
  Add : Sum
  Constant : Constant  Value=Aircraft.Control.inertia_inv_4by4  OutDataTypeStr=single
  Constant1 : Constant  Value=Aircraft.Motor.pos_m  OutDataTypeStr=single
  Constant2 : Constant  Value=Aircraft.HoverRotor.poly_thrust  OutDataTypeStr=single
  Constant3 : Constant  Value=Aircraft.HoverRotor.poly_torque  OutDataTypeStr=single
  Constant4 : Constant  Value=Aircraft.Mass.mass_kg
  Constant5 : Constant  Value=Aircraft.Mass.cg_m
  Discrete Derivative : simulink/Discrete/Discrete Derivative  gainval=1.0  ICPrevScaledInput=0.0  OutMin=[]  OutMax=[]  OutDataTypeStr=single  OutputDataTypeScalingMode=single  OutDataType=fixdt(1, 16)  OutScaling=2^-10  DoSatur=off
  Discrete Derivative1 : simulink/Discrete/Discrete Derivative  gainval=1.0  ICPrevScaledInput=0.0  OutMin=[]  OutMax=[]  OutDataTypeStr=single  OutputDataTypeScalingMode=single  OutDataType=fixdt(1, 16)  OutScaling=2^-10  DoSatur=off
  Gain : Gain  Gain=Aircraft.Control.Hover.body_rates_gain  OutDataTypeStr=single
  LowPass Filter : Subsystem
      settings: PortSchema="{\"entries\":[{\"content\":{\"sides\":[{\"content\":{\"connectorIds\":[\"Out1\"]},\"type\":\"ConnectorPlacement.EquallySpacedRectSide\",\"uuid\":\"91cc3e13-2b14-472d-8884-d1975898cd34\"},{\"content\":{\"connectorIds\":[\"In1\"],\"side\":\"RIGHT\"},\"type\":\"ConnectorPlacement.EquallySpacedRectSide\",\"uuid\":\"ce6b3021-6e32-4737-8c8e-25014706d3dd\"},{\"content\":{\"side\":\"TOP\"},\"type\":\"ConnectorPlacement.EquallySpacedRectSide\",\"uuid\":\"ad734f0b-b067-43e6-a641-0e0955250a7f\"},{\"content\":{\"side\":\"BOTTOM\"},\"type\":\"ConnectorPlacement.EquallySpacedRectSide\",\"uuid\":\"618c62c8-d4e2-4678-9fe1-905e2f147d5d\"}]},\"type\":\"ConnectorPlacement.EquallySpacedConnector\",\"uuid\":\"c0097053-d36a-473a-84fb-0616f69f4bc5\"}],\"packageUris\":[\"http://schema.mathworks.com/mf0/Connector/R2020b\"],\"version\":\"1.0\"}"
  LowPass Filter1 : Subsystem
      settings: PortSchema="{\"entries\":[{\"content\":{\"sides\":[{\"content\":{\"connectorIds\":[\"Out1\"]},\"type\":\"ConnectorPlacement.EquallySpacedRectSide\",\"uuid\":\"91cc3e13-2b14-472d-8884-d1975898cd34\"},{\"content\":{\"connectorIds\":[\"In1\"],\"side\":\"RIGHT\"},\"type\":\"ConnectorPlacement.EquallySpacedRectSide\",\"uuid\":\"ce6b3021-6e32-4737-8c8e-25014706d3dd\"},{\"content\":{\"side\":\"TOP\"},\"type\":\"ConnectorPlacement.EquallySpacedRectSide\",\"uuid\":\"ad734f0b-b067-43e6-a641-0e0955250a7f\"},{\"content\":{\"side\":\"BOTTOM\"},\"type\":\"ConnectorPlacement.EquallySpacedRectSide\",\"uuid\":\"618c62c8-d4e2-4678-9fe1-905e2f147d5d\"}]},\"type\":\"ConnectorPlacement.EquallySpacedConnector\",\"uuid\":\"c0097053-d36a-473a-84fb-0616f69f4bc5\"}],\"packageUris\":[\"http://schema.mathworks.com/mf0/Connector/R2020b\"],\"version\":\"1.0\"}"
  MATLAB Function : MATLAB Function  TreatAsAtomicUnit=on
  MATLAB Function1 : MATLAB Function  TreatAsAtomicUnit=on
  Mux : Mux  Inputs=2
  Mux1 : Mux  Inputs=2
  Saturation : Saturate  UpperLimit=1  LowerLimit=0.2
  Selector : Selector  InputPortWidth=3  IndexOptions=Index vector (dialog)  Indices=3  OutputSizes=1
  Sum : Sum  Inputs=|+-  OutDataTypeStr=single
  motor_cmds_out : Outport
  wires:
  Constant2/1 -> MATLAB Function1/3(thrust_coefs)
  MATLAB Function/1(motor_cmds) -> Add/1
  uvw_body/1 -> Selector/1
  Discrete Derivative1/1 -> MATLAB Function/2(x_ref_rate)
  Sum/1 -> Gain/1  "x_error"
  Constant4/1 -> MATLAB Function1/1(mass)
  Constant3/1 -> MATLAB Function1/4(torque_coefs)
  pqr_ref/1 -> Mux/1
  pqr/1 -> Mux1/1
  Constant1/1 -> MATLAB Function1/5(motor_pos)
  Mux1/1 -> Sum/2, Discrete Derivative/1  "x"
  Constant/1 -> MATLAB Function1/6(new_inertia_inv)
  MATLAB Function1/1(B0_mat) -> MATLAB Function/1(B0_mat)
  Gain/1 -> MATLAB Function/3(Kp_term)
  Constant5/1 -> MATLAB Function1/2(cg_pos)
  Add/1 -> LowPass Filter/1(raw_val)
  Selector/1 -> Mux1/2  "w"
  w_ref/1 -> Mux/2
  LowPass Filter1/1(filtered_val) -> Discrete Derivative1/1, Sum/1  "x_ref"
  Discrete Derivative/1 -> MATLAB Function/4(x_rate)
  Mux/1 -> LowPass Filter1/1(raw_val)  "x_ref"
  Saturation/1 -> motor_cmds_out/1
  LowPass Filter/1(filtered_val) -> Saturation/1
  prev_motor_cmds/1 -> Add/2, MATLAB Function1/7(motor_cmds)

== system quadplane_control_conf/Hover Outer Loop/Altitude Control ==
  rpy : Inport
  alt_cmd : Inport  Port=2
  alt : Inport  Port=3
  Gain : Gain  Gain=-1
  Gain1 : Gain  Gain=Aircraft.Control.Hover.alt_gain
  MATLAB Function : MATLAB Function  TreatAsAtomicUnit=on
  Saturation : Saturate  UpperLimit=Aircraft.Control.Hover.body_vert_limits(1)  LowerLimit=Aircraft.Control.Hover.body_vert_limits(2)
  Saturation1 : Saturate  UpperLimit=Aircraft.Control.Hover.nav_vert_limits(1)  LowerLimit=Aircraft.Control.Hover.nav_vert_limits(2)
  Sum : Sum  Inputs=|+-
  w_cmd : Outport
  wires:
  Gain/1 -> Saturation1/1
  alt/1 -> Sum/2
  alt_cmd/1 -> Sum/1
  Sum/1 -> Gain1/1
  Gain1/1 -> Gain/1
  rpy/1 -> MATLAB Function/1(roll_pitch)
  Saturation/1 -> w_cmd/1
  MATLAB Function/1(w_ref) -> Saturation/1
  Saturation1/1 -> MATLAB Function/2(z_dot_nav_ref)

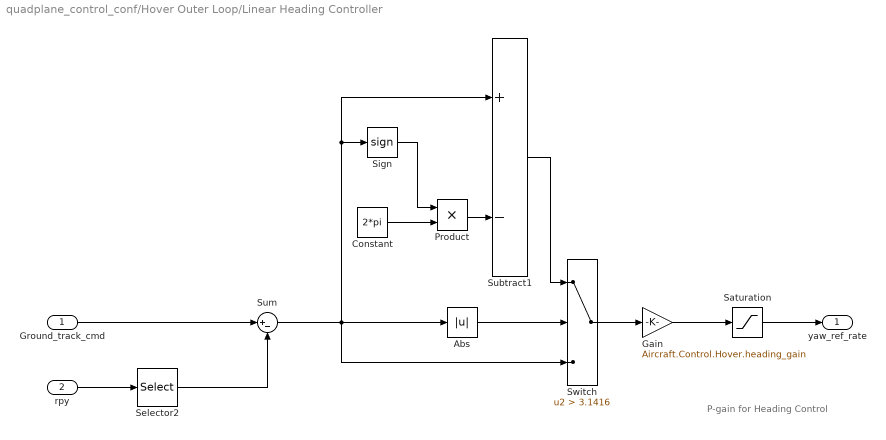
== system quadplane_control_conf/Hover Outer Loop/Linear Heading Controller ==
  note: P-gain for Heading Control
  Ground_track_cmd : Inport
  rpy : Inport  Port=2
  Abs : Abs  SaturateOnIntegerOverflow=off
  Constant : Constant  Value=2*pi  OutDataTypeStr=single
  Gain : Gain  Gain=Aircraft.Control.Hover.heading_gain
  Product : Product
  Saturation : Saturate  UpperLimit=Aircraft.Control.Hover.yaw_rate_ref_limit  LowerLimit=-Aircraft.Control.Hover.yaw_rate_ref_limit  OutDataTypeStr=single
  Selector2 : Selector  InputPortWidth=3  IndexOptions=Index vector (dialog)  Indices=3  OutputSizes=1
  Sign : Signum
  Subtract1 : Sum  Inputs=+-
  Sum : Sum  Inputs=|+-
  Switch : Switch  Criteria=u2 > Threshold  Threshold=3.1416  SaturateOnIntegerOverflow=off  InputSameDT=off
  yaw_ref_rate : Outport
  wires:
  Ground_track_cmd/1 -> Sum/1
  rpy/1 -> Selector2/1
  Selector2/1 -> Sum/2
  Gain/1 -> Saturation/1
  Saturation/1 -> yaw_ref_rate/1
  Switch/1 -> Gain/1
  Constant/1 -> Product/2
  Sum/1 -> Abs/1, Switch/3, Subtract1/1, Sign/1
  Product/1 -> Subtract1/2
  Abs/1 -> Switch/2
  Sign/1 -> Product/1
  Subtract1/1 -> Switch/1

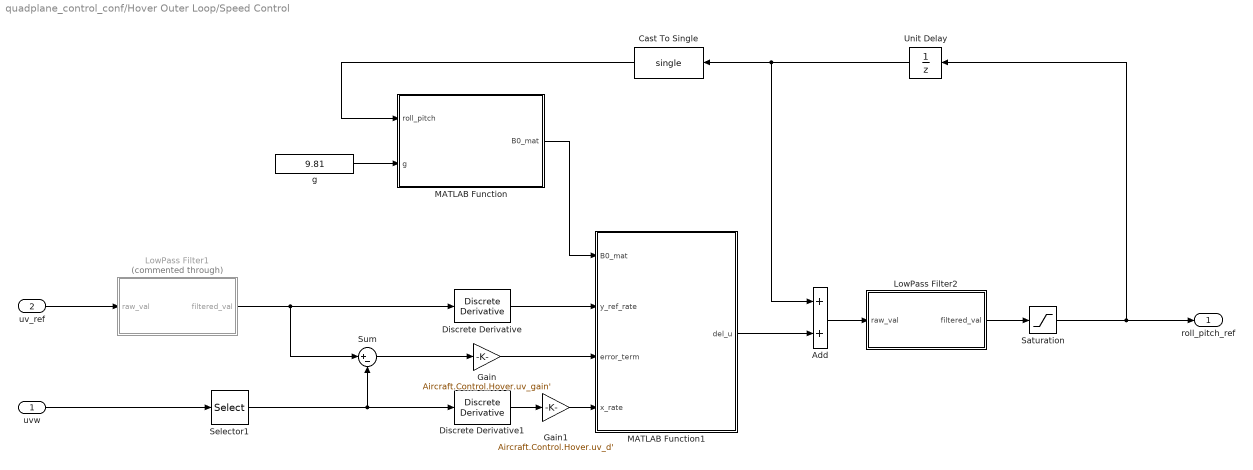
== system quadplane_control_conf/Hover Outer Loop/Speed Control ==
  uvw : Inport
  uv_ref : Inport  Port=2
  Add : Sum
  Cast To Single : DataTypeConversion  OutDataTypeStr=single  SaturateOnIntegerOverflow=off  RndMeth=Floor
  Discrete Derivative : simulink/Discrete/Discrete Derivative  gainval=1.0  ICPrevScaledInput=0.0  OutMin=[]  OutMax=[]  OutDataType=fixdt(1, 16)  OutScaling=2^-10  DoSatur=off
  Discrete Derivative1 : simulink/Discrete/Discrete Derivative  gainval=1.0  ICPrevScaledInput=0.0  OutMin=[]  OutMax=[]  OutDataType=fixdt(1, 16)  OutScaling=2^-10  DoSatur=off
  Gain : Gain  Gain=Aircraft.Control.Hover.uv_gain'
  Gain1 : Gain  Gain=Aircraft.Control.Hover.uv_d'
  LowPass Filter1 : Subsystem  Commented=through
      settings: PortSchema="{\"entries\":[{\"content\":{\"sides\":[{\"content\":{\"connectorIds\":[\"Out1\"]},\"type\":\"ConnectorPlacement.EquallySpacedRectSide\",\"uuid\":\"91cc3e13-2b14-472d-8884-d1975898cd34\"},{\"content\":{\"connectorIds\":[\"In1\"],\"side\":\"RIGHT\"},\"type\":\"ConnectorPlacement.EquallySpacedRectSide\",\"uuid\":\"ce6b3021-6e32-4737-8c8e-25014706d3dd\"},{\"content\":{\"side\":\"TOP\"},\"type\":\"ConnectorPlacement.EquallySpacedRectSide\",\"uuid\":\"ad734f0b-b067-43e6-a641-0e0955250a7f\"},{\"content\":{\"side\":\"BOTTOM\"},\"type\":\"ConnectorPlacement.EquallySpacedRectSide\",\"uuid\":\"618c62c8-d4e2-4678-9fe1-905e2f147d5d\"}]},\"type\":\"ConnectorPlacement.EquallySpacedConnector\",\"uuid\":\"c0097053-d36a-473a-84fb-0616f69f4bc5\"}],\"packageUris\":[\"http://schema.mathworks.com/mf0/Connector/R2020b\"],\"version\":\"1.0\"}"
  LowPass Filter2 : Subsystem
      settings: PortSchema="{\"entries\":[{\"content\":{\"sides\":[{\"content\":{\"connectorIds\":[\"Out1\"]},\"type\":\"ConnectorPlacement.EquallySpacedRectSide\",\"uuid\":\"91cc3e13-2b14-472d-8884-d1975898cd34\"},{\"content\":{\"connectorIds\":[\"In1\"],\"side\":\"RIGHT\"},\"type\":\"ConnectorPlacement.EquallySpacedRectSide\",\"uuid\":\"ce6b3021-6e32-4737-8c8e-25014706d3dd\"},{\"content\":{\"side\":\"TOP\"},\"type\":\"ConnectorPlacement.EquallySpacedRectSide\",\"uuid\":\"ad734f0b-b067-43e6-a641-0e0955250a7f\"},{\"content\":{\"side\":\"BOTTOM\"},\"type\":\"ConnectorPlacement.EquallySpacedRectSide\",\"uuid\":\"618c62c8-d4e2-4678-9fe1-905e2f147d5d\"}]},\"type\":\"ConnectorPlacement.EquallySpacedConnector\",\"uuid\":\"c0097053-d36a-473a-84fb-0616f69f4bc5\"}],\"packageUris\":[\"http://schema.mathworks.com/mf0/Connector/R2020b\"],\"version\":\"1.0\"}"
  MATLAB Function : MATLAB Function  TreatAsAtomicUnit=on
  MATLAB Function1 : MATLAB Function  TreatAsAtomicUnit=on
  Saturation : Saturate  UpperLimit=Aircraft.Control.Hover.roll_pitch_ref_limits'  LowerLimit=-Aircraft.Control.Hover.roll_pitch_ref_limits'
  Selector1 : Selector  InputPortWidth=3  IndexOptions=Index vector (dialog)  Indices=[1 2]  OutputSizes=1
  Sum : Sum  Inputs=|+-
  Unit Delay : UnitDelay  SampleTime=-1  HasFrameUpgradeWarning=on
  g : Constant  Value=9.81  OutDataTypeStr=single
  roll_pitch_ref : Outport
  wires:
  Saturation/1 -> Unit Delay/1, roll_pitch_ref/1
  g/1 -> MATLAB Function/2(g)
  uvw/1 -> Selector1/1
  Selector1/1 -> Discrete Derivative1/1, Sum/2
  Sum/1 -> Gain/1
  Gain/1 -> MATLAB Function1/3(error_term)
  MATLAB Function/1(B0_mat) -> MATLAB Function1/1(B0_mat)
  MATLAB Function1/1(del_u) -> Add/2
  Unit Delay/1 -> Add/1, Cast To Single/1
  Add/1 -> LowPass Filter2/1(raw_val)
  Discrete Derivative1/1 -> Gain1/1
  Gain1/1 -> MATLAB Function1/4(x_rate)
  Cast To Single/1 -> MATLAB Function/1(roll_pitch)
  Discrete Derivative/1 -> MATLAB Function1/2(y_ref_rate)
  LowPass Filter2/1(filtered_val) -> Saturation/1
  LowPass Filter1/1(filtered_val) -> Sum/1, Discrete Derivative/1
  uv_ref/1 -> LowPass Filter1/1(raw_val)

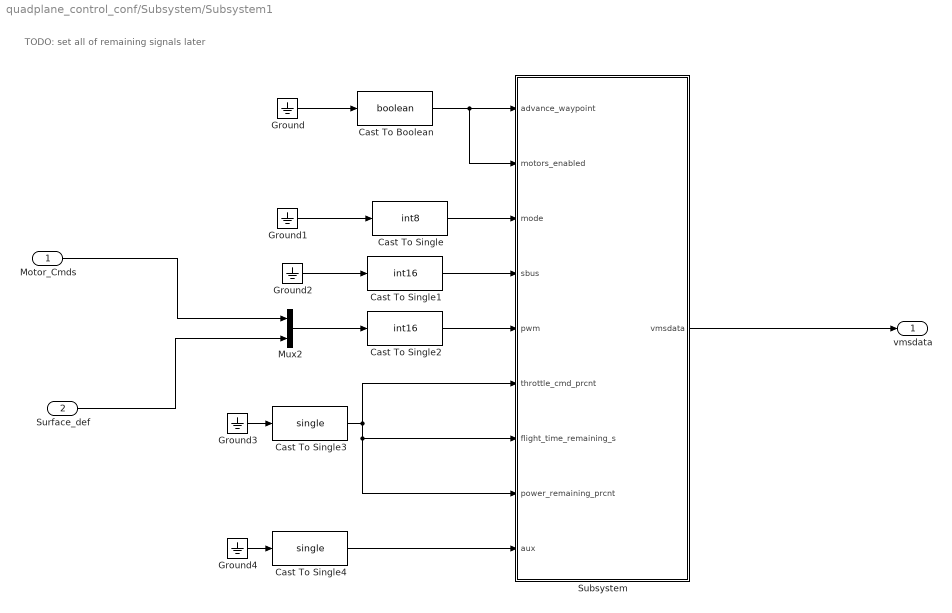
== system quadplane_control_conf/Subsystem/Subsystem1 ==
  note: TODO: set all of remaining signals later
  Motor_Cmds : Inport
  Surface_def : Inport  Port=2
  Cast To Boolean : DataTypeConversion  OutDataTypeStr=boolean  SaturateOnIntegerOverflow=off  RndMeth=Floor
  Cast To Single : DataTypeConversion  OutDataTypeStr=int8  SaturateOnIntegerOverflow=off  RndMeth=Floor
  Cast To Single1 : DataTypeConversion  OutDataTypeStr=int16  SaturateOnIntegerOverflow=off  RndMeth=Floor
  Cast To Single2 : DataTypeConversion  OutDataTypeStr=int16  SaturateOnIntegerOverflow=off  RndMeth=Floor
  Cast To Single3 : DataTypeConversion  OutDataTypeStr=single  SaturateOnIntegerOverflow=off  RndMeth=Floor
  Cast To Single4 : DataTypeConversion  OutDataTypeStr=single  SaturateOnIntegerOverflow=off  RndMeth=Floor
  Ground{,1..4} (5 alike) : Ground
  Mux2 : Mux  Inputs=2
  Subsystem : Subsystem
  vmsdata : Outport
  wires:
  Cast To Single/1 -> Subsystem/3(mode)
  Ground3/1 -> Cast To Single3/1
  Motor_Cmds/1 -> Mux2/1
  Cast To Single3/1 -> Subsystem/6(throttle_cmd_prcnt), Subsystem/8(power_remaining_prcnt), Subsystem/7(flight_time_remaining_s)
  Ground2/1 -> Cast To Single1/1
  Ground1/1 -> Cast To Single/1
  Cast To Single2/1 -> Subsystem/5(pwm)
  Cast To Single1/1 -> Subsystem/4(sbus)
  Surface_def/1 -> Mux2/2
  Cast To Single4/1 -> Subsystem/9(aux)
  Ground4/1 -> Cast To Single4/1
  Subsystem/1(vmsdata) -> vmsdata/1
  Ground/1 -> Cast To Boolean/1
  Cast To Boolean/1 -> Subsystem/2(motors_enabled), Subsystem/1(advance_waypoint)
  Mux2/1 -> Cast To Single2/1

== system quadplane_control_conf/Subsystem/deflections_PWM_denormalize ==
  note: Remap to PWM signal
  normalized_input : Inport
  Constant : Constant  Value=Aircraft.Surf.Limit.neg_deg(1)  OutDataTypeStr=single
  Constant1 : Constant  Value=1100  OutDataTypeStr=single
  Constant2 : Constant  Value=1950  OutDataTypeStr=single
  Constant3 : Constant  Value=Aircraft.Surf.Limit.pos_deg(1)  OutDataTypeStr=single
  remap : MATLAB Function  TreatAsAtomicUnit=on
  raw_output : Outport
  wires:
  Constant2/1 -> remap/5(out_max)
  Constant1/1 -> remap/4(out_min)
  Constant3/1 -> remap/3(in_max)
  Constant/1 -> remap/2(in_min)
  remap/1(raw_out) -> raw_output/1
  normalized_input/1 -> remap/1(norm_in)

== system quadplane_control_conf/Subsystem/motor_PWM_denormalize ==
  note: Remap to PWM signal
  normalized_input : Inport
  Constant : Constant  Value=0  OutDataTypeStr=single
  Constant1 : Constant  Value=1100  OutDataTypeStr=single
  Constant2 : Constant  Value=1950  OutDataTypeStr=single
  Constant3 : Constant  OutDataTypeStr=single
  remap : MATLAB Function  TreatAsAtomicUnit=on
  raw_output : Outport
  wires:
  Constant2/1 -> remap/5(out_max)
  Constant1/1 -> remap/4(out_min)
  Constant3/1 -> remap/3(in_max)
  Constant/1 -> remap/2(in_min)
  remap/1(raw_out) -> raw_output/1
  normalized_input/1 -> remap/1(norm_in)

== system quadplane_control_conf/Trajectory Command/Subsystem ==
  Mux : Mux  Inputs=2
  Step4 : Step  Time=73  After=3  OutDataTypeStr=single  SampleTime=0
  Step5 : Step  Time=27  After=0  OutDataTypeStr=single  SampleTime=0
  uv_ref_hover : Outport
  wires:
  Step5/1 -> Mux/1
  Mux/1 -> uv_ref_hover/1
  Step4/1 -> Mux/2

== system quadplane_control_conf/Trajectory Command/Subsystem1 ==
  Add3 : Sum  Inputs=++++
  Constant3 : Constant  Value=0.3  OutDataTypeStr=single
  Step3 : Step  Time=2  After=-0.8  OutDataTypeStr=single  SampleTime=0
  Step7 : Step  Time=14  Before=-0.8  After=0.5  OutDataTypeStr=single  SampleTime=0
  Step8 : Step  Time=25  Before=0.5  After=2.75  OutDataTypeStr=single  SampleTime=0
  hdg_cmd : Outport
  wires:
  Step7/1 -> Add3/2
  Step8/1 -> Add3/4
  Constant3/1 -> Add3/3
  Add3/1 -> hdg_cmd/1
  Step3/1 -> Add3/1

== system quadplane_control_conf/Trajectory Command/Subsystem2 ==
  mode_input : Inport
  Constant : Constant  Value=0  OutDataTypeStr=single
  Ramp1 : simulink/Sources/Ramp  slope=Aircraft.Control.modes.hover2forward_airspeed_ramp  start=7  InitialOutput=0
  Ramp2 : simulink/Sources/Ramp  slope=Aircraft.Control.modes.forward2hover_airspeed_ramp  start=52  InitialOutput=0
  Saturation1 : Saturate  UpperLimit=22  LowerLimit=0  OutDataTypeStr=single
  Saturation2 : Saturate  UpperLimit=22  LowerLimit=0  OutDataTypeStr=single
  Scope4 : Scope
  Sum : Sum  Inputs=|++
  Switch : Switch  Criteria=u2 > Threshold  SaturateOnIntegerOverflow=off  InputSameDT=off
  airspeed_cmd : Outport
  wires:
  Ramp1/1 -> Saturation1/1
  Constant/1 -> Switch/3
  Ramp2/1 -> Sum/2
  Saturation2/1 -> Switch/1, Scope4/1
  Sum/1 -> Saturation2/1
  Saturation1/1 -> Sum/1
  mode_input/1 -> Switch/2
  Switch/1 -> airspeed_cmd/1

== system quadplane_control_conf/Trajectory Command/Subsystem3 ==
  Add2 : Sum  Inputs=+++
  Constant2 : Constant  Value=-110  OutDataTypeStr=single
  Step1 : Step  Time=15  Before=100  After=110  OutDataTypeStr=single  SampleTime=0
  Step2 : Step  Time=40  Before=110  After=90  OutDataTypeStr=single  SampleTime=0
  altitude_cmd : Outport
  wires:
  Add2/1 -> altitude_cmd/1
  Step2/1 -> Add2/2
  Constant2/1 -> Add2/3
  Step1/1 -> Add2/1
